simulink model "energy_consume_test2"  (R2023a)
settings: Solver=VariableStepAuto  StartTime=0.0  StopTime=50  RelTol=1e-3
libraries: spsIdealSwitchLib x6, spsSeriesRLCBranchLib x5, spsGroundLib x4, spsBreakerLib x3, spsParallelRLCBranchLib x3, spsStairGeneratorLib x3, spsDCVoltageSourceLib x2, spsDCMachineLib x1, spspowerguiLib x1, spsVoltageMeasurementLib x1
settings Model: Creator=ASUS  LastModifiedBy=ASUS

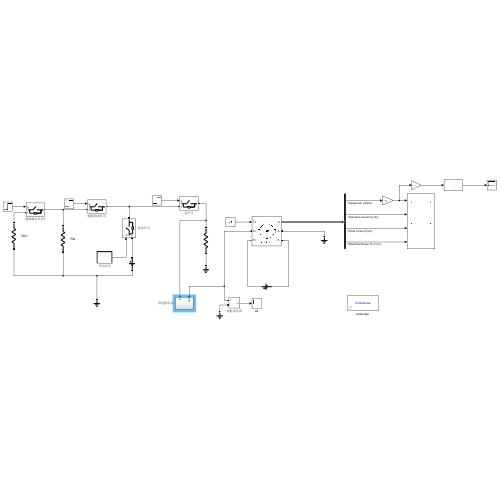
[thumbnail: Simulink's stored preview of the top-level diagram]
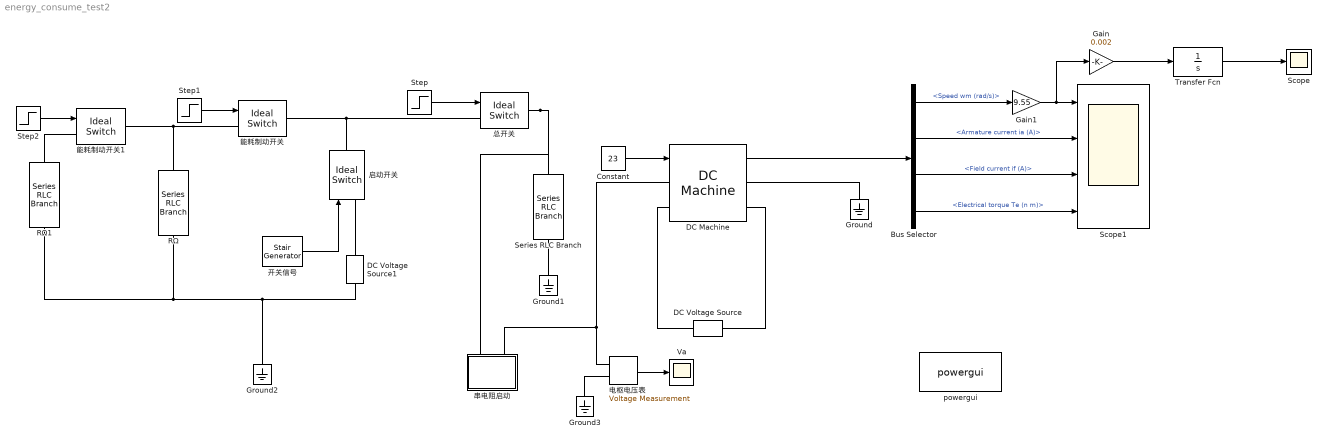
== system energy_consume_test2 ==
  Bus Selector : BusSelector  OutputSignals=Speed wm (rad/s),Armature current ia (A),Field current if (A),Electrical torque Te (n m)
  Constant : Constant  Value=23
  DC Machine : spsDCMachineLib/DC Machine  PresetModel=No  MechanicalLoad=Torque TL  FieldType=Wound  ShowDetailedParameters=on  MeasurementBus=off  RLa=[1.5 0.03]  RLf=[20 100]  Laf=0.1116  MachineConstant=Torque constant (N.m/A)  Ke=1.8  Kt=1.8  J=0.02215  Bm=0.002953  Tf=0.5161  w0=1  Ifinit=11  TsPowergui=0  TsBlock=-1
  DC Voltage Source : spsDCVoltageSourceLib/DC Voltage Source  Amplitude=220  Measurements=None
  DC Voltage Source1 : spsDCVoltageSourceLib/DC Voltage Source  Amplitude=220  Measurements=None
  Gain : Gain  Gain=0.002
  Gain1 : Gain  Gain=9.55
  Ground{,1..3} (4 alike) : spsGroundLib/Ground  LConnTagsString=a
  RΩ : spsSeriesRLCBranchLib/Series RLC Branch  LConnTagsString=__new0  RConnTagsString=__new0  BranchType=R  Resistance=0.575  Inductance=1e-3  SetiL0=off  InitialCurrent=0  Capacitance=1e-6  Setx0=off  InitialVoltage=0  Measurements=None
  RΩ1 : spsSeriesRLCBranchLib/Series RLC Branch  LConnTagsString=__new0  RConnTagsString=__new0  BranchType=R  Resistance=0.1  Inductance=1e-3  SetiL0=off  InitialCurrent=0  Capacitance=1e-6  Setx0=off  InitialVoltage=0  Measurements=None
  Scope : Scope
  Scope1 : Scope  NumInputPorts=4
  Series RLC Branch : spsSeriesRLCBranchLib/Series RLC Branch  LConnTagsString=__new0  RConnTagsString=__new0  BranchType=R  Resistance=10000  Inductance=1e-3  SetiL0=off  InitialCurrent=0  Capacitance=1e-6  Setx0=off  InitialVoltage=0  Measurements=None
  Step : Step  Time=0.0001  SampleTime=0
  Step1 : Step  Time=11.5  SampleTime=0
  Step2 : Step  Time=20  SampleTime=0
  Transfer Fcn : TransferFcn  Denominator=[1 0]
  Va : Scope
  powergui : spspowerguiLib/powergui  Priority=1  SimulationMode=Continuous  SampleTime=50e-6  frequency=60  Iterations=50  frequencyindice=0  Pbase=100e6  ErrMax=1e-4  UnitsV=kV  UnitsW=MW  buscounter=0  FunctionMessages=off  echomessages=off  EnableUseOfTLC=off  CurrentSourceSwitches=off  DisableSnubberDevices=off  DisableRonSwitches=off  DisableVfSwitches=off  DisplayEquations=off  AutomaticDiscreteSolvers=off  SolverType=Tustin/Backward Euler (TBE)  Interpol=off  ExternalGateDelay=off  methode=off  Ts=100  x0status=blocks  SPID=on  SwTol=0  HookPort=off  NonlinearTolerance=1e-4  nMaxIteration=100  ContinueOnMaxIteration=off  RestoreLinks=warning  ResistiveCurrentMeasurement=off  Frange=[0:2:500]  Ylog=off  Xlog=on  ShowGrid=off  save=off  variable=ZData  structure=0  ZoomFFT=off  StartTime=0.0  cycles=1  DisplayStyle=1  fundamental=60  FreqAxis=off  MaxFrequency=1000  frequencyindicesteady=1  RmsSteady=1  display=off
  串电阻启动 : Subsystem
  启动开关 : spsIdealSwitchLib/Ideal Switch  Ron=0.001  Lon=0  IC=1  Rs=1e5  Cs=inf  Measurements=off
  开关信号 : spsStairGeneratorLib/Stair Generator  t=[0,0.0001,11.5]  e=[0,1,0]  Ts=0
  总开关 : spsIdealSwitchLib/Ideal Switch  Ron=0.001  Lon=0  IC=0  Rs=1e5  Cs=inf  Measurements=off
  电枢电压表 : spsVoltageMeasurementLib/Voltage Measurement  PhasorSimulation=off  OutputType=Complex  PSBequivalent=0
  能耗制动开关 : spsIdealSwitchLib/Ideal Switch  Ron=0.001  Lon=0  IC=1  Rs=1e5  Cs=inf  Measurements=off
  能耗制动开关1 : spsIdealSwitchLib/Ideal Switch  Ron=0.001  Lon=0  IC=1  Rs=1e5  Cs=inf  Measurements=off
  wires:
  开关信号/1 -> 启动开关/1
  电枢电压表/1 -> Va/1
  Gain1/1 -> Gain/1, Scope1/1
  Step/1 -> 总开关/1
  Constant/1 -> DC Machine/1
  Bus Selector/4 -> Scope1/4  "<Electrical torque Te (n m)>"
  Bus Selector/3 -> Scope1/3  "<Field current if (A)>"
  Bus Selector/1 -> Gain1/1  "<Speed wm (rad/s)>"
  DC Machine/1 -> Bus Selector/1
  Bus Selector/2 -> Scope1/2  "<Armature current ia (A)>"
  Step1/1 -> 能耗制动开关/1
  Transfer Fcn/1 -> Scope/1
  Gain/1 -> Transfer Fcn/1
  Step2/1 -> 能耗制动开关1/1
  connections:
  总开关/RConn1 -- 串电阻启动/LConn1 -- Series RLC Branch/LConn1
  能耗制动开关/RConn1 -- 启动开关/RConn1 -- 总开关/LConn1
  DC Voltage Source1/LConn1 -- Ground2/LConn1 -- RΩ1/LConn1 -- RΩ/LConn1
  DC Machine/LConn1 -- 电枢电压表/LConn1 -- 串电阻启动/LConn2
  DC Machine/RConn2 -- DC Voltage Source/LConn1
  RΩ/RConn1 -- 能耗制动开关1/RConn1 -- 能耗制动开关/LConn1
  DC Machine/RConn1 -- Ground/LConn1
  Series RLC Branch/RConn1 -- Ground1/LConn1
  启动开关/LConn1 -- DC Voltage Source1/RConn1
  DC Machine/LConn2 -- DC Voltage Source/RConn1
  电枢电压表/LConn2 -- Ground3/LConn1
  RΩ1/RConn1 -- 能耗制动开关1/LConn1

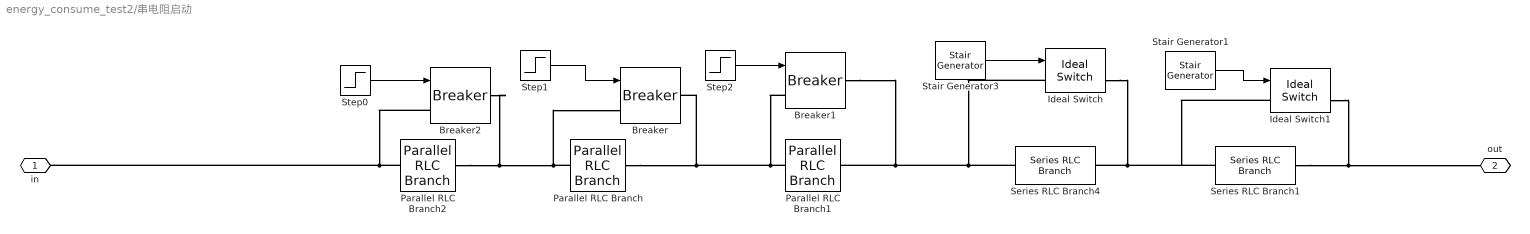
== system energy_consume_test2/串电阻启动 ==
  Breaker : spsBreakerLib/Breaker  InitialState=0  SwitchingTimes="[1/60  5/60]"  External=on  BreakerResistance=0.01  SnubberResistance=1e6  SnubberCapacitance=inf  Measurements=None  MoreParameters=on  NoBreakLoop=off
  Breaker1 : spsBreakerLib/Breaker  InitialState=0  SwitchingTimes="[1/60  5/60]"  External=on  BreakerResistance=0.01  SnubberResistance=1e6  SnubberCapacitance=inf  Measurements=None  MoreParameters=on  NoBreakLoop=off
  Breaker2 : spsBreakerLib/Breaker  InitialState=0  SwitchingTimes="[1/60  5/60]"  External=on  BreakerResistance=0.01  SnubberResistance=1e6  SnubberCapacitance=inf  Measurements=None  MoreParameters=on  NoBreakLoop=off
  Ideal Switch : spsIdealSwitchLib/Ideal Switch  Ron=0.001  Lon=0  IC=0  Rs=1e5  Cs=inf  Measurements=on
  Ideal Switch1 : spsIdealSwitchLib/Ideal Switch  Ron=0.001  Lon=0  IC=1  Rs=1e5  Cs=inf  Measurements=on
  Parallel RLC Branch : spsParallelRLCBranchLib/Parallel RLC Branch  LConnTagsString=a  RConnTagsString=__new0  BranchType=R  Resistance=1.154  Inductance=1e-3  SetiL0=off  InitialCurrent=0  Capacitance=1e-6  Setx0=off  InitialVoltage=0  Measurements=None
  Parallel RLC Branch1 : spsParallelRLCBranchLib/Parallel RLC Branch  LConnTagsString=a  RConnTagsString=__new0  BranchType=R  Resistance=1.842  Inductance=1e-3  SetiL0=off  InitialCurrent=0  Capacitance=1e-6  Setx0=off  InitialVoltage=0  Measurements=None
  Parallel RLC Branch2 : spsParallelRLCBranchLib/Parallel RLC Branch  LConnTagsString=a  RConnTagsString=__new0  BranchType=R  Resistance=0.722  Inductance=1e-3  SetiL0=off  InitialCurrent=0  Capacitance=1e-6  Setx0=off  InitialVoltage=0  Measurements=None
  Series RLC Branch1 : spsSeriesRLCBranchLib/Series RLC Branch  LConnTagsString=__new0  RConnTagsString=__new0  BranchType=R  Resistance=1  Inductance=1e-3  SetiL0=off  InitialCurrent=0  Capacitance=1e-6  Setx0=off  InitialVoltage=0  Measurements=None
  Series RLC Branch4 : spsSeriesRLCBranchLib/Series RLC Branch  LConnTagsString=__new0  RConnTagsString=__new0  BranchType=R  Resistance=3.1  Inductance=1e-3  SetiL0=off  InitialCurrent=0  Capacitance=1e-6  Setx0=off  InitialVoltage=0  Measurements=None
  Stair Generator1 : spsStairGeneratorLib/Stair Generator  t=[0 0.001 4 11.5 17]  e=[0 1 0 1 0]  Ts=0
  Stair Generator3 : spsStairGeneratorLib/Stair Generator  t=[0 0.001 4 11.5]  e=[0 1 0 1]  Ts=0
  Step0 : Step  SampleTime=0
  Step1 : Step  Time=1.5  SampleTime=0
  Step2 : Step  Time=2  SampleTime=0
  in : PMIOPort  Side=Left
  out : PMIOPort  Port=2  Side=Left
  wires:
  Step0/1 -> Breaker2/1
  Step2/1 -> Breaker1/1
  Step1/1 -> Breaker/1
  Stair Generator3/1 -> Ideal Switch/1
  Stair Generator1/1 -> Ideal Switch1/1
  connections:
  Parallel RLC Branch1/LConn1 -- Parallel RLC Branch/RConn1 -- Breaker/RConn1 -- Breaker1/LConn1
  Series RLC Branch4/LConn1 -- Ideal Switch/LConn1 -- Breaker1/RConn1 -- Parallel RLC Branch1/RConn1
  Parallel RLC Branch2/LConn1 -- in/RConn1 -- Breaker2/LConn1
  Parallel RLC Branch2/RConn1 -- Breaker2/RConn1 -- Parallel RLC Branch/LConn1 -- Breaker/LConn1
  Ideal Switch/RConn1 -- Ideal Switch1/LConn1 -- Series RLC Branch1/LConn1 -- Series RLC Branch4/RConn1
  Series RLC Branch1/RConn1 -- Ideal Switch1/RConn1 -- out/RConn1
